simulink model "clik_inverse"  (R2022b)
settings: Solver=ode1  StartTime=0.0  StopTime=4  FixedStep=0.001  RelTol=1e-3
undefined symbols (not defined in the file or in its folder): DiscIntNeverNeededParam, q0, Tc
settings Model: Creator=Xp  LastModifiedBy=reube
settings SolverCC: AlgebraicLoopSolver=TrustRegion
settings DataIOCC: LimitDataPoints=on  SaveFormat=Array  SignalLoggingSaveFormat=ModelDataLogs  ReturnWorkspaceOutputs=off
settings OptimizationCC: ExpressionDepthLimit=2147483647  InitFltsAndDblsToZero=on  LifeSpan=inf
settings DebuggingCC: SaveWithParameterizedLinksMsg=none  UnderspecifiedInitializationDetection=Classic  MergeDetectMultiDrivingBlocksExec=none  SolverPrmCheckMsg=warning  MultiTaskDSMMsg=warning  MultiTaskCondExecSysMsg=none  FcnCallInpInsideContextMsg=warning  UnconnectedInputMsg=warning  UnconnectedOutputMsg=warning  UnconnectedLineMsg=warning  StateNameClashWarn=warning  SFUnexpectedBacktrackingDiag=warning  SFNoUnconditionalDefaultTransitionDiag=warning  SFExecutionAtInitializationDiag=none  SFMachineParentedDataDiag=warning  ArithmeticOperatorsInVariantConditions=warning
settings HardwareCC: ProdBitPerPointer=32  ProdBitPerSizeT=32  ProdBitPerPtrDiffT=32  ProdLargestAtomicFloat=None  ProdIntDivRoundTo=Undefined  ProdEndianess=Unspecified  ProdWordSize=32  ProdHWDeviceType=32-bit Generic
settings ModelReferenceCC: EnableRefExpFcnMdlSchedulingChecks=on  PropagateSignalLabelsOutOfModel=off
settings SFSimCC: CustomCodeUndefinedFunction=UseInterfaceOnly
settings RTWCC: DLArmComputeVersion=19.05
settings CodeAppCC: StateflowObjectComments=on
settings GRTTargetCC: TargetLangStandard=C89/C90 (ANSI)  CombineOutputUpdateFcns=off  GRTInterface=on
settings ConfigComp: CovMetricSettings=dw  CovSaveCumulativeToWorkspaceVar=on  CovSaveSingleToWorkspaceVar=on

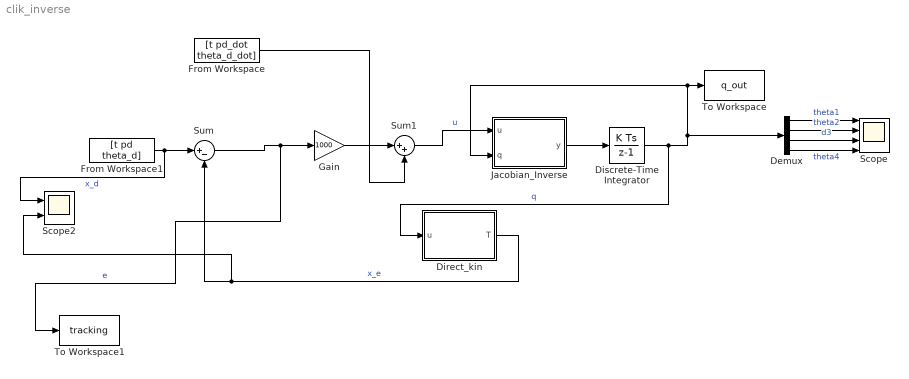
== system clik_inverse ==
  Demux : Demux
  Direct_kin : MATLAB Function  TreatAsAtomicUnit=on
  Discrete-Time Integrator : DiscreteIntegrator  InitialCondition=q0  SampleTime=Tc  LimitOutput=on  UpperSaturationLimit=[pi/2;pi/4;1;2*pi]  LowerSaturationLimit=[-pi/2;-pi/2;0.25;-2*pi]  ICPrevOutput=DiscIntNeverNeededParam  ICPrevScaledInput=DiscIntNeverNeededParam
  From Workspace : FromWorkspace  VariableName=[t pd_dot theta_d_dot]  SampleTime=Tc
  From Workspace1 : FromWorkspace  VariableName=[t pd theta_d]  SampleTime=Tc
  Gain : Gain  Gain=1000
  Jacobian_Inverse : MATLAB Function  TreatAsAtomicUnit=on
  Scope : Scope  NumInputPorts=4
  Scope2 : Scope  NumInputPorts=2
  Sum : Sum  Inputs=|+-
  Sum1 : Sum  Inputs=|++
  To Workspace : ToWorkspace  VariableName=q_out  SampleTime=-1
  To Workspace1 : ToWorkspace  VariableName=tracking  SampleTime=Tc
  wires:
  Demux/4 -> Scope/4  "theta4"
  Demux/2 -> Scope/2  "theta2"
  Sum/1 -> To Workspace1/1, Gain/1  "e"
  Discrete-Time Integrator/1 -> Direct_kin/1(u), Demux/1, Jacobian_Inverse/2(q), To Workspace/1  "q"
  From Workspace/1 -> Sum1/2
  From Workspace1/1 -> Scope2/1, Sum/1  "x_d"
  Demux/1 -> Scope/1  "theta1"
  Demux/3 -> Scope/3  "d3"
  Gain/1 -> Sum1/1
  Jacobian_Inverse/1(y) -> Discrete-Time Integrator/1
  Direct_kin/1(T) -> Scope2/2, Sum/2  "x_e"
  Sum1/1 -> Jacobian_Inverse/1(u)  "u"

== matlab function clik_inverse/Jacobian_Inverse ==
  data: u input; y output; q input
function y = fcn(u,q)
y=zeros(4,1);

Jac= jacobian_inverse(q)


y = (Jac)* u;

end

== matlab function clik_inverse/Direct_kin ==
  data: u input; T output
function T = fcn(u)
       T=direct_kin(u)
end
